simulink model "APP_Plaus12"  (R2016b)
settings: configuration reference "CodeGenConfigSet" (kept outside this file)
values from neighbouring files (symbols this model uses):
  APP_PlaAPPDefDeb_C = Calibration.Parameter    [init_APP_Plaus12.m]
  APP_PlaAPPDefOK_C = Calibration.Parameter    [init_APP_Plaus12.m]
  APP_uSyncMin_C = Calibration.Parameter    [init_APP_Plaus12.m]
  MoFAPP_dRawSigFac_C = Calibration.Parameter    [init_APP_Plaus12.m]
  MoFAPP_uSync_CUR = Calibration.Parameter    [init_APP_Plaus12.m]
  MoFAPP_uSync_CURX = Calibration.Parameter    [init_APP_Plaus12.m]
undefined symbols (not defined in the file or in its folder): APP_Plaus12_DT
libraries: CXLib x3
settings Model: Creator=lenovo  LastModifiedBy=wangrui
settings ConfigSetRef: SourceLocation=Base Workspace

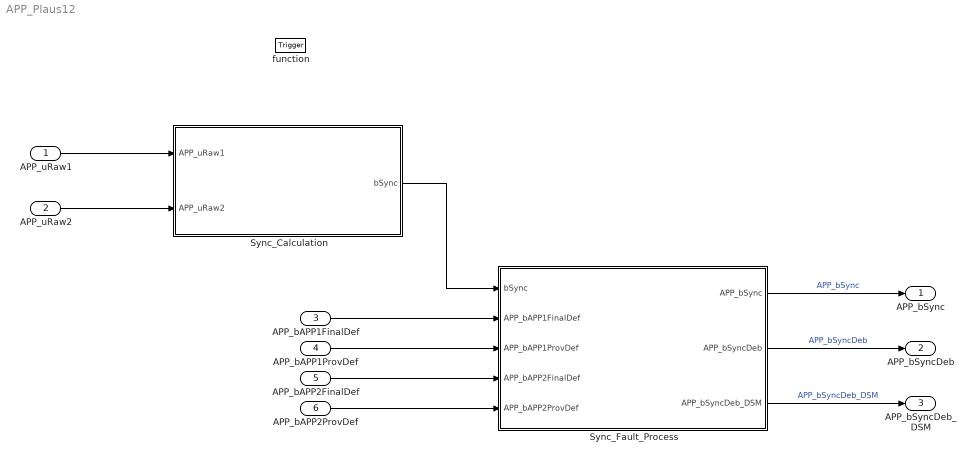
== system APP_Plaus12 ==
  APP_uRaw1 : Inport  Tag=mv  Description=Acceleration Pedal Position D  OutMin=0  OutMax=5000  OutDataTypeStr=Ad_mv
  APP_uRaw2 : Inport  Tag=mv  Description=Acceleration Pedal Position E  Port=2  OutMin=0  OutMax=5000  OutDataTypeStr=Ad_mv
  APP_bAPP1FinalDef : Inport  Description=Status Sensor 1 of the acceleration pedal finally defect  Port=3  OutMin=0  OutMax=1  OutDataTypeStr=boolean
  APP_bAPP1ProvDef : Inport  Description=Status Sensor 1 of the acceleration pedal temporary defect  Port=4  OutMin=0  OutMax=1  OutDataTypeStr=boolean
  APP_bAPP2FinalDef : Inport  Description=Status Sensor 2 of the acceleration pedal finally defect  Port=5  OutMin=0  OutMax=1  OutDataTypeStr=boolean
  APP_bAPP2ProvDef : Inport  Description=Status Sensor 2 of the acceleration pedal temporary defect  Port=6  OutMin=0  OutMax=1  OutDataTypeStr=boolean
  function : TriggerPort  TriggerType=function-call  VariantControl=Variant
  Sync_Calculation : Subsystem
  Sync_Fault_Process : Subsystem
  APP_bSync : Outport  Description=Status temporary sync check  OutMin=0  OutMax=1  OutDataTypeStr=boolean
  APP_bSyncDeb : Outport  Description=Status debounced sync check  Port=2  OutMin=0  OutMax=1  OutDataTypeStr=boolean
  APP_bSyncDeb_DSM : Outport  Description=Status debounced sync check finally defect  Port=3  OutMin=0  OutMax=1  OutDataTypeStr=boolean
  wires:
  APP_uRaw2/1 -> Sync_Calculation/2(APP_uRaw2)
  APP_uRaw1/1 -> Sync_Calculation/1(APP_uRaw1)
  Sync_Calculation/1(bSync) -> Sync_Fault_Process/1(bSync)
  APP_bAPP1FinalDef/1 -> Sync_Fault_Process/2(APP_bAPP1FinalDef)
  APP_bAPP1ProvDef/1 -> Sync_Fault_Process/3(APP_bAPP1ProvDef)
  APP_bAPP2FinalDef/1 -> Sync_Fault_Process/4(APP_bAPP2FinalDef)
  APP_bAPP2ProvDef/1 -> Sync_Fault_Process/5(APP_bAPP2ProvDef)
  Sync_Fault_Process/1(APP_bSync) -> APP_bSync/1  "APP_bSync"
  Sync_Fault_Process/2(APP_bSyncDeb) -> APP_bSyncDeb/1  "APP_bSyncDeb"
  Sync_Fault_Process/3(APP_bSyncDeb_DSM) -> APP_bSyncDeb_DSM/1  "APP_bSyncDeb_DSM"

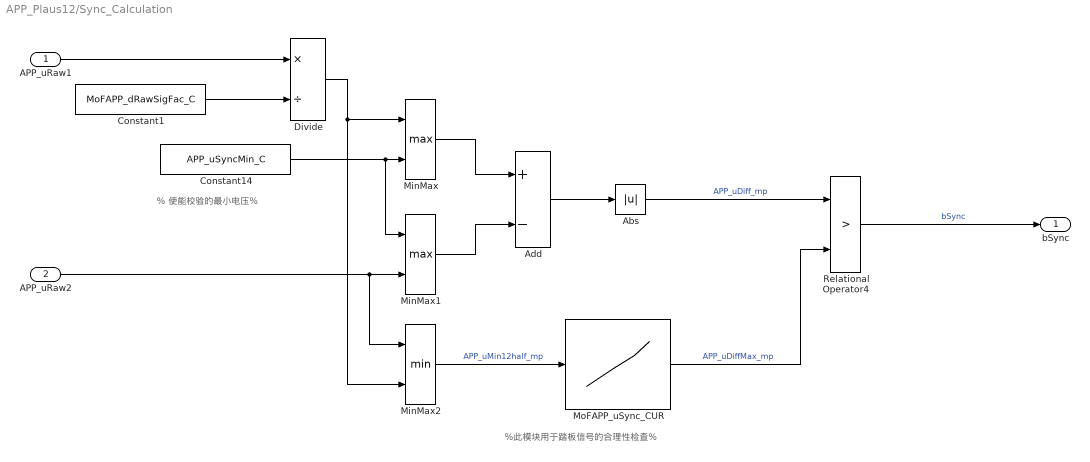
== system APP_Plaus12/Sync_Calculation ==
  note: %此模块用于踏板信号的合理性检查%
  note: % 使能校验的最小电压%
  APP_uRaw1 : Inport
  APP_uRaw2 : Inport  Port=2
  Abs : Abs  OutDataTypeStr=Inherit: Inherit via back propagation
  Add : Sum  Inputs=+-  InputSameDT=on
  Constant1 : Constant  Value=MoFAPP_dRawSigFac_C  SampleTime=-1
  Constant14 : Constant  Value=APP_uSyncMin_C  SampleTime=-1
  Divide : Product  Inputs=*/  OutDataTypeStr=Ad_mv
  MinMax : MinMax  Function=max  Inputs=2  InputSameDT=on
  MinMax1 : MinMax  Function=max  Inputs=2  InputSameDT=on
  MinMax2 : MinMax  Inputs=2  InputSameDT=on
  MoFAPP_uSync_CUR : Lookup_n-D  NumberOfTableDimensions=1  BreakpointsForDimension1=MoFAPP_uSync_CURX  IndexSearchMethod=Linear search  BeginIndexSearchUsingPreviousIndexResult=on  Table=MoFAPP_uSync_CUR  ExtrapMethod=Clip  UseLastTableValue=on  InternalRulePriority=Speed  OutDataTypeStr=Inherit: Inherit via back propagation  SaturateOnIntegerOverflow=on  MaximumIndicesForEachDimension=MoFAPP_uSync_CURMAX
  Relational Operator4 : RelationalOperator  Operator=>  OutDataTypeStr=boolean  RndMeth=Nearest  InputSameDT=on
  bSync : Outport
  wires:
  Relational Operator4/1 -> bSync/1  "bSync"
  MinMax2/1 -> MoFAPP_uSync_CUR/1  "APP_uMin12half_mp"
  MinMax1/1 -> Add/2
  Divide/1 -> MinMax/1, MinMax2/2
  MinMax/1 -> Add/1
  APP_uRaw2/1 -> MinMax1/2, MinMax2/1
  Abs/1 -> Relational Operator4/1  "APP_uDiff_mp"
  Constant14/1 -> MinMax/2, MinMax1/1
  APP_uRaw1/1 -> Divide/1
  MoFAPP_uSync_CUR/1 -> Relational Operator4/2  "APP_uDiffMax_mp"
  Constant1/1 -> Divide/2
  Add/1 -> Abs/1

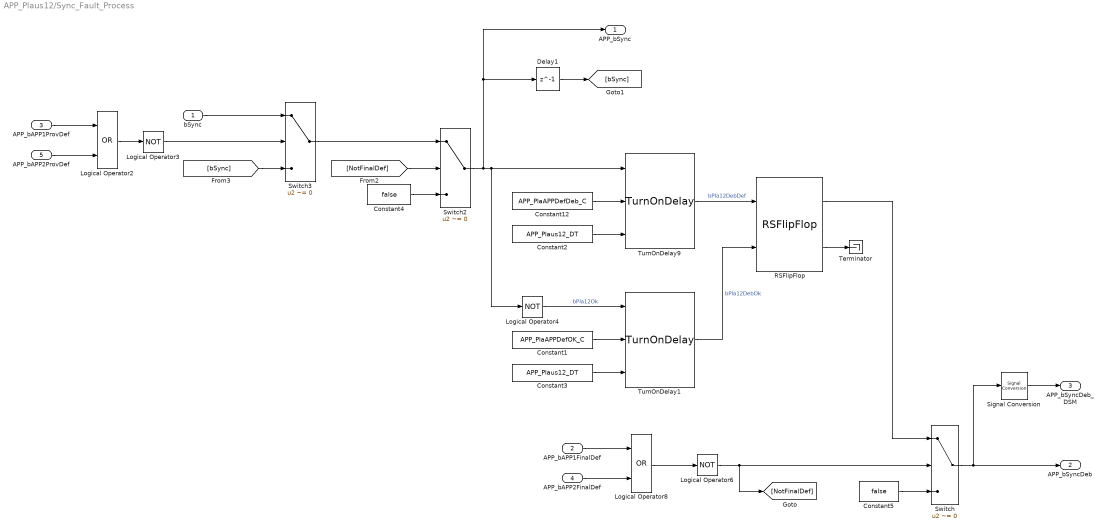
== system APP_Plaus12/Sync_Fault_Process ==
  bSync : Inport
  APP_bAPP1FinalDef : Inport  Tag=-  Description=Status Sensor 1 of the acceleration pedal finally defect  Port=2  OutMin=0  OutMax=1  OutDataTypeStr=boolean
  APP_bAPP1ProvDef : Inport  Tag=-  Description=Status Sensor 1 of the acceleration pedal temporary defect  Port=3  OutMin=0  OutMax=1  OutDataTypeStr=boolean
  APP_bAPP2FinalDef : Inport  Tag=-  Description=Status Sensor 2 of the acceleration pedal finally defect  Port=4  OutMin=0  OutMax=1  OutDataTypeStr=boolean
  APP_bAPP2ProvDef : Inport  Tag=-  Description=Status Sensor 2 of the acceleration pedal temporary defect  Port=5  OutMin=0  OutMax=1  OutDataTypeStr=boolean
  Constant1 : Constant  Value=APP_PlaAPPDefOK_C
  Constant12 : Constant  Value=APP_PlaAPPDefDeb_C
  Constant2 : Constant  Value=APP_Plaus12_DT  OutDataTypeStr=Inherit: Inherit via back propagation
  Constant3 : Constant  Value=APP_Plaus12_DT  OutDataTypeStr=Inherit: Inherit via back propagation
  Constant4 : Constant  Value=false  OutDataTypeStr=boolean
  Constant5 : Constant  Value=false  OutDataTypeStr=boolean
  Delay1 : Delay  DelayLength=1  InitialCondition=0  StateName=time
  Logical Operator2 : Logic  Operator=OR  OutDataTypeStr=boolean
  Logical Operator3 : Logic  Operator=NOT  AllPortsSameDT=off  OutDataTypeStr=boolean
  Logical Operator4 : Logic  Operator=NOT  AllPortsSameDT=off  OutDataTypeStr=boolean
  Logical Operator6 : Logic  Operator=NOT  AllPortsSameDT=off  OutDataTypeStr=boolean
  Logical Operator8 : Logic  Operator=OR  OutDataTypeStr=boolean
  RSFlipFlop : CXLib/RSFlipFlop
  Signal Conversion : SignalConversion  OverrideOpt=off
  Switch : Switch  Criteria=u2 ~= 0  InputSameDT=on
  Switch2 : Switch  Criteria=u2 ~= 0  InputSameDT=on
  Switch3 : Switch  Criteria=u2 ~= 0  InputSameDT=on
  Terminator : Terminator
  TurnOnDelay1 : CXLib/TurnOnDelay
  TurnOnDelay9 : CXLib/TurnOnDelay
  APP_bSync : Outport  Tag=-  Description=Status temporary sync check  OutMin=0  OutMax=1  OutDataTypeStr=boolean
  APP_bSyncDeb : Outport  Tag=-  Description=Status debounced sync check  Port=2  OutMin=0  OutMax=1  OutDataTypeStr=boolean
  APP_bSyncDeb_DSM : Outport  Tag=-  Description=Status debounced sync check  Port=3  OutMin=0  OutMax=1  OutDataTypeStr=boolean
  wires:
  bSync/1 -> Switch3/1
  Delay1/1 -> [bSync]
  RSFlipFlop/1 -> Switch/1
  Logical Operator2/1 -> Logical Operator3/1
  Constant5/1 -> Switch/3
  Logical Operator8/1 -> Logical Operator6/1
  APP_bAPP2ProvDef/1 -> Logical Operator2/2
  APP_bAPP2FinalDef/1 -> Logical Operator8/2
  APP_bAPP1FinalDef/1 -> Logical Operator8/1
  Logical Operator6/1 -> Switch/2, [NotFinalDef]
  APP_bAPP1ProvDef/1 -> Logical Operator2/1
  [NotFinalDef] -> Switch2/2
  Switch3/1 -> Switch2/1
  Constant4/1 -> Switch2/3
  Switch/1 -> APP_bSyncDeb/1, Signal Conversion/1
  Logical Operator3/1 -> Switch3/2
  Signal Conversion/1 -> APP_bSyncDeb_DSM/1
  Constant3/1 -> TurnOnDelay1/3
  Constant2/1 -> TurnOnDelay9/3
  RSFlipFlop/2 -> Terminator/1
  Switch2/1 -> TurnOnDelay9/1, Logical Operator4/1, Delay1/1, APP_bSync/1
  Logical Operator4/1 -> TurnOnDelay1/1  "bPla12Ok"
  TurnOnDelay1/1 -> RSFlipFlop/2  "bPla12DebOk"
  Constant1/1 -> TurnOnDelay1/2
  Constant12/1 -> TurnOnDelay9/2
  TurnOnDelay9/1 -> RSFlipFlop/1  "bPla12DebDef"
  [bSync] -> Switch3/3
